simulink model "robot"  (R2018a)
settings: Solver=VariableStepAuto  StartTime=0.0  StopTime=20  RelTol=1e-3
InitFcn:
  | robot_
values from neighbouring files (symbols this model uses):
  ki = kt(1,3)    [control_nolineal_linealizacion_entrada_estado.m]    (also in e_mimo.m; ej_mimo.m = kt(:,2+1:end); ej_mimo2.m = kt(:,2+1:end); ejemplo_2.m)
  kp = kt(1,1:2)    [control_nolineal_linealizacion_entrada_estado.m]    (also in e_mimo.m; ej_mimo.m = kt(:,1:2); ej_mimo2.m = kt(:,1:2); ejemplo_2.m)
libraries: simulink x1
settings Model: Creator=carma  LastModifiedBy=carma

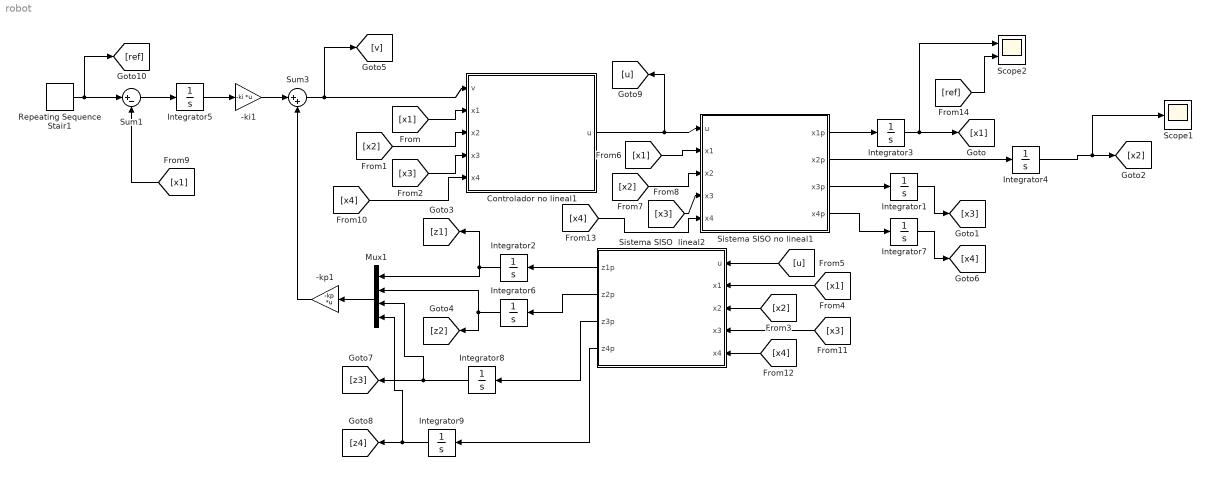
== system robot ==
  -ki1 : Gain  Gain=-ki  Multiplication=Matrix(K*u) (u vector)
  -kp1 : Gain  Gain=-kp  Multiplication=Matrix(K*u) (u vector)
  Controlador no lineal1 : MATLAB Function  TreatAsAtomicUnit=on
  Integrator{1..9} (9 alike) : Integrator
  Mux1 : Mux
  Repeating Sequence Stair1 : simulink/Sources/Repeating Sequence Stair  OutValues=[0.6 0.4 -0.2 0.1 -0.3].'  tsamp=1.5  OutMin=[]  OutMax=[]  OutDataTypeStr=double  OutputDataTypeScalingMode=double  OutDataType=fixdt(0,8)  ConRadixGroup=Best Precision: Vector-wise  OutScaling=2^-12
  Scope1 : Scope
  Scope2 : Scope  NumInputPorts=2
  Sistema SISO  lineal2 : MATLAB Function  TreatAsAtomicUnit=on
  Sistema SISO no lineal1 : MATLAB Function  TreatAsAtomicUnit=on
  Sum1 : Sum  Inputs=|+-
  Sum3 : Sum  Inputs=|++
  wires:
  Sum3/1 -> [v], Controlador no lineal1/1(v)
  Sistema SISO no lineal1/2(x2p) -> Integrator4/1
  Sum1/1 -> Integrator5/1
  Controlador no lineal1/1(u) -> [u], Sistema SISO no lineal1/1(u)
  Sistema SISO no lineal1/1(x1p) -> Integrator3/1
  Mux1/1 -> -kp1/1
  Integrator5/1 -> -ki1/1
  -ki1/1 -> Sum3/1
  -kp1/1 -> Sum3/2
  Sistema SISO no lineal1/3(x3p) -> Integrator1/1
  [x1] -> Controlador no lineal1/2(x1)
  [x3] -> Controlador no lineal1/4(x3)
  [x2] -> Controlador no lineal1/3(x2)
  Integrator1/1 -> [x3]
  Integrator4/1 -> [x2], Scope1/1
  Sistema SISO  lineal2/1(z1p) -> Integrator2/1
  Integrator2/1 -> Mux1/1, [z1]
  Integrator6/1 -> [z2], Mux1/2
  Sistema SISO  lineal2/2(z2p) -> Integrator6/1
  [x1] -> Sistema SISO  lineal2/2(x1)
  [x2] -> Sistema SISO  lineal2/3(x2)
  [u] -> Sistema SISO  lineal2/1(u)
  Integrator3/1 -> Scope2/1, [x1]
  [x3] -> Sistema SISO no lineal1/4(x3)
  [x2] -> Sistema SISO no lineal1/3(x2)
  [x1] -> Sistema SISO no lineal1/2(x1)
  [x1] -> Sum1/2
  Sistema SISO no lineal1/4(x4p) -> Integrator7/1
  Integrator7/1 -> [x4]
  [x4] -> Controlador no lineal1/5(x4)
  Integrator8/1 -> Mux1/3, [z3]
  Sistema SISO  lineal2/3(z3p) -> Integrator8/1
  Sistema SISO  lineal2/4(z4p) -> Integrator9/1
  Integrator9/1 -> Mux1/4, [z4]
  [x3] -> Sistema SISO  lineal2/4(x3)
  [x4] -> Sistema SISO  lineal2/5(x4)
  [x4] -> Sistema SISO no lineal1/5(x4)
  Repeating Sequence Stair1/1 -> [ref], Sum1/1
  [ref] -> Scope2/2

== matlab function robot/Sistema SISO  lineal2 ==
  data: u input; z1p output; x1 input; x2 input; z2p output; x3 input; x4 input; z3p output; z4p output
function [z1p,z2p,z3p,z4p]= fcn(u,x1,x2,x3,x4)

%parametros
M=5;
g=9.8;
L=0.3;
k=3;
J=2;
I=1.5;


% 
% x1p=x2;
% x2p=-(M*g*L/I)*sin(x1)-k/I*(x1-x3);
% x3p=x4;
% x4p=(k/J)*(x1-x3)+u/J;

z1p=x2;
z2p=-(M*g*L/I)*sin(x1)-k/I*(x1-x3);
z3p=-(M*g*L/I)*x2*cos(x1)-(k/I)*(x2-x4);
a=(M*g*L/I)*sin(x1)*(x2^2+(M*g*L/I)*cos(x1)+k/I)+(k/I)*(x1-x3)*(k/I+k/J+(M*g*L/I)*cos(x1));
z4p=(k/(I*J))*u+a;


% z1p=z2;
% z2p=z3;
% z3p=z4;
% z4p=v;

%s=5;
%syms y
%Cx3=(2+10^(pk2-y))/(1+10^(pk2-y)+10^(pk1+pk2-2*y));
%h=-x1+x2-x3*Cx3+10^(-y)-10^(y-pkw)==0;

%s=double(solve(h));

== matlab function robot/Controlador no lineal1 ==
  data: v input; u output; x1 input; x2 input; x3 input; x4 input
function u = fcn(v,x1,x2,x3,x4)

%parametros
M=5;
g=9.8;
L=0.3;
k=3;
J=2;
I=1.5;

a=(M*g*L/I)*sin(x1)*(x2^2+(M*g*L/I)*cos(x1)+k/I)+(k/I)*(x1-x3)*(k/I+k/J+(M*g*L/I)*cos(x1));
u=(I*J/k)*(v-a);

%s=5;
%syms y
%Cx3=(2+10^(pk2-y))/(1+10^(pk2-y)+10^(pk1+pk2-2*y));
%h=-x1+x2-x3*Cx3+10^(-y)-10^(y-pkw)==0;

%s=double(solve(h));

== matlab function robot/Sistema SISO no lineal1 ==
  data: u input; x1p output; x1 input; x2 input; x2p output; x3 input; x3p output; x4 input; x4p output
function [x1p,x2p,x3p,x4p]= fcn(u,x1,x2,x3,x4)

%parametros
M=5;
g=9.8;
L=0.3;
k=3;
J=2;
I=1.5;



x1p=x2;
x2p=-(M*g*L/I)*sin(x1)-(k/I)*(x1-x3);
x3p=x4;
x4p=(k/J)*(x1-x3)+u/J;

%s=5;
%syms y
%Cx3=(2+10^(pk2-y))/(1+10^(pk2-y)+10^(pk1+pk2-2*y));
%h=-x1+x2-x3*Cx3+10^(-y)-10^(y-pkw)==0;

%s=double(solve(h));
